simulink model "mogen_SMU_test"  (Simulink 9.2)
settings: Solver=ode4  StartTime=0.0  StopTime=6  FixedStep=model_sample_time  RelTol=1e-3
undefined symbols (not defined in the file): magnitude, model_sample_time
libraries: utils x4, simulink x2
(part 2 of 3)

== matlab function move2pose1/p2p/Cartesian_ipol2/rotation/Embedded MATLAB Function1 ==
  data: t input double; qd output double; s0 input double; v0 input double; sf input double; vm input double; am input double; dqd output double; ddqd output double; ipol_finished output double; T_scale input double; interpoly input double
function [qd,dqd,ddqd, ipol_finished] = calc_qd(t,s0,v0,sf,vm,am,T_scale,interpoly)
% This function calculates a one dimensional movement with a trapezodial 
% signal for velocity over time. Additionally it is able to adapt to shifts
% in the maximum allowed velocity.
%
% Inputs:
% t         current runtime
% s0        start value for motion in position
% v0        start value for motion in velocity
% sf        final value for motion in position
% vm        maximum allowed velocity
% am        maximum allowed acceleration
% T_scale   Scaling factor for duration of adaption
% interpoly Which interpolation to use
%
% Outputs:
% qd        disered position at current time
% dqd       disered velocity at current time
% ddqd      disered acceleration at current time
% ipol_finished 
%           motion is finished

%% Initialize persistent variables for adaption motion
persistent vm1 adpt ti qi qf T t_shift
if isempty(vm1)
    vm1 = vm;       %remembers the max velocity from last run
end
if isempty(adpt)
    adpt = false;   %stores if an adaption motion is activated
end
if isempty(ti)
    ti = 0;         %Initial time step for adaption motion
end
if isempty(qi)
    qi = zeros(3,1);%Initial values (pos,vel,acc) for adaption motion
end
if isempty(qf)
    qf = zeros(3,1);%Final values (pos,vel,acc) for adaption motion
end
if isempty(T)
    T = 0;          %Duration of adaption motion; tf = ti+T
end
if isempty(t_shift)
    t_shift = 0;    %Time distance with which the current reference motion is shifted
end

%% This If runs only for one timestep!!!
% If current max velocity is unequal to old one 
% Not directly at the beginning
% Dont start new while a adaption is still running, to prevent reset of
%   initial values
if abs(vm-vm1)>1e-3 && t>0.001 && adpt==false                       
    adpt=true;          % Activate adaption
    ti=t;               % Set initial timestep to current step

    %%% inital set of position, velo, acceleration for adaption motion 
    % is the same as the old mogen would do (t_shift is not updated at
    % this time!)
    [qi, ~] = interpolator(ti+t_shift, compute_traj_parameters(s0, v0, sf, vm1, am));

    %%% computes the time shift for shifting the new motion to the end
    % point of the old motion. So at which time the new motion has
    % the same qd? Then calculate the time distance to the inital
    % time of the change in velocities
    % t_shift < 0 if new motion is faster (vm>vm1)
    % t_shift > 0 if new motion is slower (vm<vm1)
    % interpolator_1 is the inverse function of interpolator!
    t_shift = interpolator_1(qi(1), compute_traj_parameters(s0, v0, sf, vm, am)) - ti ;

    %%% Additional shift for adaption motion = Duration of adaption motion 
    switch interpoly
        case 0
            T=0;
            adpt=false;         %no adatption  
        case 1
            T = (vm/am)*1.5;    %tanhlog
        case 2
            T = (pi*abs(qi(2)-vm))/(2*am);  %Cosine version
        case 3
            T = (vm/am);        %poly3
        case 4
            T = 1.5*(abs(qi(2)-vm)/am); %poly4
        case 5
            T = (vm/am);        %poly5 
        otherwise
            T = (vm/am);        %rest
    end

    % Scale Duration if needed
    T = T*T_scale;

    %%% The additional shift for adaption motion is dependent on the
    % difference in the velocities. See report for details.
    t_shift  = t_shift+(T/2)*((vm1/vm)-1);

    %%% Calculate final values for adaption motion. Which are reached
    % at inital time plus duration of adaption and new time shift
    [qf, ~] = interpolator(ti+T+t_shift, compute_traj_parameters(s0, v0, sf, vm, am));

end

%% Here the actual motion is calculated
% Interpolates the values of pos,vel,acc (qv) with parameters and current time t    
[qdv, ipol_finished] =interpolator(t+t_shift, compute_traj_parameters(s0, v0, sf, vm, am));  

%% If adaption motion needed
if adpt == true 

    %%% calculate the adaption moition, which takes time from ti to
    % ti+T. t is the current runtime, _i initial values, _f final
    % values, _m maximum values

    switch interpoly
        case 0
            adpt=false;                             %no adatption  
        case 1
            qdv = tanhlog(t,ti,T,qi,qf,vm,am);      %tanhlog
        case 2
            qdv = cosine(t,ti,T,qi,qf,vm,am);       %Cosine version
        case 3
            qdv = poly3(t,ti,T,qi,qf,vm,am);        %poly3
        case 4
            qdv = poly4(t,ti,T,qi,qf,vm,am);        %poly4
        case 5
            qdv = poly5(t,ti,T,qi,qf,vm,am);        %poly5 
        case 6
            qdv = poly6(t,ti,T,qi,qf,vm,am);        %poly6 
        case 7
            qdv = poly4_mean(t,ti,T,qi,qf,vm,am);   %poly4_mean 
        case 8
            qdv = poly5_2mean(t,ti,T,qi,qf,vm,am);  %poly5_2mean 
        case 9
            qdv = tanhmean(t,ti,T,qi,qf,vm,am);     %tanhmean 
        otherwise
            error('Unknown adaption motion');       %rest
    end

    %if time is equal than the finish time => adaption motion is complete
    %But it is aborted one timestep earlier, since the finish timestep
    %is already computed correctly by the standard interpolator.
    if t>=(ti+T-0.001)  %Has to be finished a bit earlier, due to errors at end
        adpt=false;     %If adaption finished => reset
    end
end

%% Set output
if sf==s0          % No motion needed if start = end 
    qd = s0;       % => set initial values
    dqd = v0;
    ddqd= 0;  
else     
    qd = qdv(1);   % set output
    dqd = qdv(2);
    ddqd = qdv(3);        
end

vm1 = vm;  %remember current max velocity

end

function [qv] = poly3(t,ti,T,qvi,qvf,dqm,ddqm)
%POLY3 computes a polynomial trajectory of degree 3 between initial (_i) 
%values and final (_f) values of position q, velocity dq and accelerataion
%ddq. Taken from Melchiorri presentation page 19

qi = qvi(1);      %split input vectors in pos,vel,acc
dqi = qvi(2);
ddqi = qvi(3);
qf = qvf(1);
dqf = qvf(2);
ddqf = qvf(3);
      
% current duration of motion dt
dt = t-ti;                      

% compute coefficients
a0 = qi;
a1 = dqi;
a2 = (-3*(qi-qf)-(2*dqi+dqf)*T)/(T^2);
a3 = (2*(qi-qf)+(dqi+dqf)*T)/(T^3);

% compute pos,vel,acc desired (_d)
qd = a0+a1*dt+a2*dt^2+a3*dt^3;
dqd = a1+2*a2*dt+3*a3*dt^2;
ddqd = 2*a2+6*a3*dt;

qv = [qd;dqd;ddqd]; %Send values back

end

function [qv] = poly4(t,ti,T,qvi,qvf,dqm,ddqm)
%POLY4 computes a polynomial trajectory of degree 4 between initial (_i) 
%values and final (_f) values of position q, velocity dq and accelerataion
%ddq. inspired by old function in here

qi = qvi(1);      %split input vectors in pos,vel,acc
dqi = qvi(2);
ddqi = qvi(3);
qf = qvf(1);
dqf = qvf(2);
ddqf = qvf(3);
      
% current duration of motion dt
dt = t-ti;                      

% a2 = 0;
% a3 = -4/9*ddqm^2/(dqi-dqm);
% a4 = -4/27*ddqm^3/(dqi-dqm)^2;
a2 = 0;
a3 = -4/9*ddqm^2/abs(dqi-dqf);
a4 = 4/27*ddqm^3/abs(dqi-dqf)^2;

a0 = qi;
a1 = dqi;
% a2 = 0.5*ddqi;
% a3 = (4*(qf-qi)-(dqf+3*dqi)*T-ddqi*(T^2))/(T^3);
% a4 = (3*(qi-qf)+(dqf+2*dqi)*T+0.5*ddqi*(T^2))/(T^4);

% compute pos,vel,acc desired (_d)
qd = (a4*dt^4+a3*dt^3+a2*dt^2+a1*dt+a0);
dqd = 4*a4*dt^3+3*a3*dt^2+2*a2*dt+a1;
ddqd = 12*a4*dt^2+6*a3*dt+2*a2;

qv = [qd;dqd;ddqd]; %Send values back

end

function [qv] = poly4_mean(t,ti,T,qvi,qvf,dqm,ddqm)
%POLY4 computes a polynomial trajectory of degree 4 between initial (_i) 
%values and final (_f) values of position q, velocity dq and accelerataion
%ddq with mean velocity at T/2. self made

qi = qvi(1);      %split input vectors in pos,vel,acc
dqi = qvi(2);
ddqi = qvi(3);
qf = qvf(1);
dqf = qvf(2);
ddqf = qvf(3);
      
% current duration of motion dt
dt = t-ti;                     

b = [qi dqi qf dqf 0.5*(dqi+dqf)]';

M_inv = [...
       1,     0,      0,          0,           0;
       0,     1,      0,          0,           0;
   6/T^2,  -2/T, -6/T^2,    5/(4*T),    27/(4*T);
 -16/T^3, 1/T^2, 16/T^3, -7/(2*T^2), -27/(2*T^2);
   9/T^4,     0, -9/T^4,  9/(4*T^3),  27/(4*T^3)];

a = M_inv * b;

% compute pos,vel,acc desired (_d)

qd = a(1)+a(2)*dt+a(3)*dt^2+a(4)*dt^3+a(5)*dt^4;
dqd = a(2)+2*a(3)*dt+3*a(4)*dt^2+4*a(5)*dt^3;
ddqd = 2*a(3)+6*a(4)*dt+12*a(5)*dt^2;

qv = [qd;dqd;ddqd]; %Send values back

end

function [qv] = poly5(t,ti,T,qvi,qvf,dqm,ddqm)
%POLY5 computes a polynomial trajectory of degree 5 between initial (_i) 
%values and final (_f) values of position q, velocity dq and accelerataion
%ddq. Taken from Melchiorri presentation page 25

qi = qvi(1);      %split input vectors in pos,vel,acc
dqi = qvi(2);
ddqi = qvi(3);
qf = qvf(1);
dqf = qvf(2);
ddqf = qvf(3);
      
% current duration of motion dt
dt = t-ti;                      

% compute coefficients
a0 = qi;
a1 = dqi;
a2 = 0.5*ddqi;
a3 = (20*(qf-qi)-(8*dqf+12*dqi)*T-(3*ddqf-ddqi)*T^2)/(2*T^3);
a4 = (30*(qi-qf)+(14*dqf+16*dqi)*T+(3*ddqf-2*ddqi)*T^2)/(2*T^4);
a5 = (12*(qf-qi)-6*(dqf+dqi)*T-(ddqf-ddqi)*T^2)/(2*T^5);

% compute pos,vel,acc desired (_d)
qd = a0+a1*dt+a2*dt^2+a3*dt^3+a4*dt^4+a5*dt^5;
dqd = a1+2*a2*dt+3*a3*dt^2+4*a4*dt^3+5*a5*dt^4;
ddqd = 2*a2+6*a3*dt+12*a4*dt^2+20*a5*dt^3;

qv = [qd;dqd;ddqd]; %Send values back

end

function [qv] = poly5_2mean(t,ti,T,qvi,qvf,dqm,ddqm)
%POLY5 computes a polynomial trajectory of degree 5 between initial (_i) 
%values and final (_f) values of position q, velocity dq and accelerataion
%ddq with 2*mean steps at T/3 and 2T/3. self made

qi = qvi(1);      %split input vectors in pos,vel,acc
dqi = qvi(2);
ddqi = qvi(3);
qf = qvf(1);
dqf = qvf(2);
ddqf = qvf(3);
      
% current duration of motion dt
dt = t-ti;                      

% compute coefficients
b = [qi dqi qf dqf 0.5*(dqi+dqf)+(1/6)*(dqi-dqf) 0.5*(dqi+dqf)+(1/6)*(dqi-dqf)]';

M_inv = [...
        1,          0,        0,           0,            0,           0;
        0,          1,        0,           0,            0,           0;
  -30/T^2,  -13/(2*T),   30/T^2,   -13/(4*T),    -27/(4*T),   -27/(2*T);
  110/T^3, 67/(4*T^2), -110/T^3,  49/(4*T^2),  135/(4*T^2), 189/(4*T^2);
 -135/T^4,    -18/T^3,  135/T^4, -63/(4*T^3), -189/(4*T^3),     -54/T^3;
   54/T^5, 27/(4*T^4),  -54/T^5,  27/(4*T^4),   81/(4*T^4),  81/(4*T^4)];

a = M_inv * b;

% compute pos,vel,acc desired (_d)

qd = a(1)+a(2)*dt+a(3)*dt^2+a(4)*dt^3+a(5)*dt^4+a(6)*dt^5;
dqd = a(2)+2*a(3)*dt+3*a(4)*dt^2+4*a(5)*dt^3+5*a(6)*dt^4;
ddqd = 2*a(3)+6*a(4)*dt+12*a(5)*dt^2+20*a(6)*dt^3;

qv = [qd;dqd;ddqd]; %Send values back

end

function [qv] = poly6(t,ti,T,qvi,qvf,dqm,ddqm)
%POLY6 computes a polynomial trajectory of degree 6 between initial (_i) 
%values and final (_f) values of position q, velocity dq and accelerataion
%ddq with mean velocity at T/3. self made

qi = qvi(1);      %split input vectors in pos,vel,acc
dqi = qvi(2);
ddqi = qvi(3);
qf = qvf(1);
dqf = qvf(2);
ddqf = qvf(3);

% current duration of motion dt
dt = t-ti;                      

% compute coefficients
b = [qi dqi 0.5*ddqi qf dqf ddqf 0.5*(dqi+dqf)]';

M_inv = [...
       1,      0,      0,       0,           0,          0,            0;
       0,      1,      0,       0,           0,          0,            0;
       0,      0,      1,       0,           0,          0,            0;
  20/T^3, -6/T^2,   -4/T, -20/T^3,  23/(4*T^2),   -1/(2*T),   81/(4*T^2);
 -75/T^4,  8/T^3,  6/T^2,  75/T^4, -89/(4*T^3),      2/T^2, -243/(4*T^3);
  84/T^5, -3/T^4, -4/T^3, -84/T^5, 105/(4*T^4), -5/(2*T^3),  243/(4*T^4);
 -30/T^6,      0,  1/T^4,  30/T^6, -39/(4*T^5),      1/T^4,  -81/(4*T^5)];

a = M_inv * b;

% compute pos,vel,acc desired (_d)

qd = a(1)+a(2)*dt+a(3)*dt^2+a(4)*dt^3+a(5)*dt^4+a(6)*dt^5+a(7)*dt^6;
dqd = a(2)+2*a(3)*dt+3*a(4)*dt^2+4*a(5)*dt^3+5*a(6)*dt^4+6*a(7)*dt^5;
ddqd = 2*a(3)+6*a(4)*dt+12*a(5)*dt^2+20*a(6)*dt^3+30*a(7)*dt^4;

qv = [qd;dqd;ddqd]; %Send values back

end

function [qv] = cosine(t,ti,T,qvi,qvf,dqm,ddqm)
%COSINE computes a cosine trajectory between initial (_i) 
%values and final (_f) values of position q, velocity dq and accelerataion
%ddq with respect to the maximum values (_m). t is the current runtime

qi = qvi(1);      %split input vectors in pos,vel,acc
dqi = qvi(2);
ddqi = qvi(3);
qf = qvf(1);
dqf = qvf(2);
ddqf = qvf(3);
      
% often needed values

%T = (pi*abs(dqf-dqi))/(2*ddqm); % total duration of motion T (with am)
%T = abs((2*(qf-qi))/(dqi-dqf));
dt = t-ti;                      % current duration of motion dt

%cm = (T/(2*pi))*(dqm-(1/T)*(qf-qi));
c = qi-0.5*(dqi+dqf)*ti;
%cn = qf-0.5*(dqi+dqf)*(ti+T);
%c = cn + 0.5*(1+cos((pi/T)*dt))*(ca-cn);


% if t<(ti+(T/2))
%     c = qi - 0.5*(dqi+dqf)*ti;
% else
%     c = qf - 0.5*(((dqi+dqf)/2)+dqf)*tf;
% end

%c = (qi+qf)/2 - 0.5*(dqi+dqf)*(ti+(T/2)) - 0.5*(dqi-dqf)*(T/pi);
% compute pos,vel,acc desired (_d)
%qd = qi + (1/T)*(qf-qi)*dt + cm*sin(((2*pi)/T)*dt);
qd = 0.5*(dqi+dqf)*t + 0.5*(T/pi)*(dqi-dqf)*sin((pi/T)*dt) + c;
dqd = 0.5*(dqi+dqf) + 0.5*(dqi-dqf)*cos((pi/T)*dt);
ddqd = -0.5*(pi/T)*(dqi-dqf)*sin((pi/T)*dt);

qv = [qd;dqd;ddqd]; %Send values back

end

function [qv] = tanhmean(t,ti,T,qvi,qvf,dqm,ddqm)
%TANHMEAN computes a tanh trajectory between initial (_i) 
%values and final (_f) values of position q, velocity dq and accelerataion
%ddq with respect to the maximum values (_m). t is the current runtime
%selfmade

qi = qvi(1);      %split input vectors in pos,vel,acc
dqi = qvi(2);
ddqi = qvi(3);
qf = qvf(1);
dqf = qvf(2);
ddqf = qvf(3);
      
% current duration of motion dt
dt = t-ti;                      
t_norm = dt/T;
theta = 4;

qd = 0.5*(1/theta)*(dqf-dqi)*log(cosh(theta*(t_norm-0.5))) ...
     + 0.5*(dqi+dqf)*t_norm ...
     + qf - 0.5*(1/theta)*(dqf-dqi)*log(cosh(0.5*theta));
     %+ qi - 0.5*(1/theta)*(dqf-dqi)*log(cosh(-0.5*theta));
dqd = 0.5*(dqi+dqf) + 0.5*(dqf-dqi)*tanh(theta*(t_norm-0.5));
ddqd = 0.5*theta*(dqf-dqi)*sech(t_norm-0.5)^2;

qv = [qd;dqd;ddqd]; %Send values back

end

function [qv] = tanhlog(t,ti,T,qvi,qvf,dqm,ddqm)
%TANHLOG computes a tanh-log trajectory between initial (_i) 
%values and final (_f) values of position q, velocity dq and accelerataion
%ddq with respect to the maximum values (_m). t is the current runtime
%taken from Internet

qi = qvi(1);      %split input vectors in pos,vel,acc
dqi = qvi(2);
ddqi = qvi(3);
qf = qvf(1);
dqf = qvf(2);
ddqf = qvf(3);
      
% current duration of motion dt
dt = t-ti;                      

a = dqi;
b = qi;      
c = dqf;
d = qf-dqf*T;
k = d-b;

x = (a*dt+b-c*dt-d+k)/(2*k);
w = (tanh(((log(1-x))^2-(log(x))^2)/3)+1)/2;
p = tanh((log(2-x)-log(x))*(1-(1/sqrt(2))*(log(2-x)+log(x))))+2*x-1;
q = tanh((log(x+1)-log(1-x))*(1-(1/sqrt(2))*(log(1-x)+log(x+1))));
s = p*(1-w)+q*w;

qd = k*s+c*dt+d-k;
dqd=(3*((tanh(((2^(1/2)*(log((10*dt)/3) + log(2 - (10*dt)/3)))/2 - 1)*(log((10*dt)/3) - log(2 - (10*dt)/3)))^2 - 1)*(((2^(1/2)*(log((10*dt)/3) + log(2 - (10*dt)/3)))/2 - 1)*(10/(3*((10*dt)/3 - 2)) - 1/dt) - (2^(1/2)*(10/(3*((10*dt)/3 - 2)) + 1/dt)*(log((10*dt)/3) - log(2 - (10*dt)/3)))/2) + 20/3)*(tanh(log((10*dt)/3)^2/3 - log(1 - (10*dt)/3)^2/3)/2 + 1/2))/100 - (3*((2*log((10*dt)/3))/(3*dt) - (20*log(1 - (10*dt)/3))/(9*((10*dt)/3 - 1)))*(tanh(log((10*dt)/3)^2/3 - log(1 - (10*dt)/3)^2/3)^2 - 1)*((20*dt)/3 + tanh(((2^(1/2)*(log((10*dt)/3) + log(2 - (10*dt)/3)))/2 - 1)*(log((10*dt)/3) - log(2 - (10*dt)/3))) - 1))/200 + (3*(tanh(((2^(1/2)*(log(1 - (10*dt)/3) + log((10*dt)/3 + 1)))/2 - 1)*(log(1 - (10*dt)/3) - log((10*dt)/3 + 1)))^2 - 1)*((10/(3*((10*dt)/3 - 1)) - 10/(3*((10*dt)/3 + 1)))*((2^(1/2)*(log(1 - (10*dt)/3) + log((10*dt)/3 + 1)))/2 - 1) + (2^(1/2)*(10/(3*((10*dt)/3 - 1)) + 10/(3*((10*dt)/3 + 1)))*(log(1 - (10*dt)/3) - log((10*dt)/3 + 1)))/2)*(tanh(log((10*dt)/3)^2/3 - log(1 - (10*dt)/3)^2/3)/2 - 1/2))/100 + (3*tanh(((2^(1/2)*(log(1 - (10*dt)/3) + log((10*dt)/3 + 1)))/2 - 1)*(log(1 - (10*dt)/3) - log((10*dt)/3 + 1)))*((2*log((10*dt)/3))/(3*dt) - (20*log(1 - (10*dt)/3))/(9*((10*dt)/3 - 1)))*(tanh(log((10*dt)/3)^2/3 - log(1 - (10*dt)/3)^2/3)^2 - 1))/200 + 3/10;
ddqd=(3*((tanh(((2^(1/2)*(log((10*dt)/3) + log(2 - (10*dt)/3)))/2 - 1)*(log((10*dt)/3) - log(2 - (10*dt)/3)))^2 - 1)*(2^(1/2)*(10/(3*((10*dt)/3 - 2)) + 1/dt)*(10/(3*((10*dt)/3 - 2)) - 1/dt) - ((2^(1/2)*(log((10*dt)/3) + log(2 - (10*dt)/3)))/2 - 1)*(100/(9*((10*dt)/3 - 2)^2) - 1/dt^2) + (2^(1/2)*(100/(9*((10*dt)/3 - 2)^2) + 1/dt^2)*(log((10*dt)/3) - log(2 - (10*dt)/3)))/2) + 2*tanh(((2^(1/2)*(log((10*dt)/3) + log(2 - (10*dt)/3)))/2 - 1)*(log((10*dt)/3) - log(2 - (10*dt)/3)))*(tanh(((2^(1/2)*(log((10*dt)/3) + log(2 - (10*dt)/3)))/2 - 1)*(log((10*dt)/3) - log(2 - (10*dt)/3)))^2 - 1)*(((2^(1/2)*(log((10*dt)/3) + log(2 - (10*dt)/3)))/2 - 1)*(10/(3*((10*dt)/3 - 2)) - 1/dt) - (2^(1/2)*(10/(3*((10*dt)/3 - 2)) + 1/dt)*(log((10*dt)/3) - log(2 - (10*dt)/3)))/2)^2)*(tanh(log((10*dt)/3)^2/3 - log(1 - (10*dt)/3)^2/3)/2 + 1/2))/100 - (3*((2*log((10*dt)/3))/(3*dt) - (20*log(1 - (10*dt)/3))/(9*((10*dt)/3 - 1)))*((tanh(((2^(1/2)*(log((10*dt)/3) + log(2 - (10*dt)/3)))/2 - 1)*(log((10*dt)/3) - log(2 - (10*dt)/3)))^2 - 1)*(((2^(1/2)*(log((10*dt)/3) + log(2 - (10*dt)/3)))/2 - 1)*(10/(3*((10*dt)/3 - 2)) - 1/dt) - (2^(1/2)*(10/(3*((10*dt)/3 - 2)) + 1/dt)*(log((10*dt)/3) - log(2 - (10*dt)/3)))/2) + 20/3)*(tanh(log((10*dt)/3)^2/3 - log(1 - (10*dt)/3)^2/3)^2 - 1))/100 + (3*(tanh(log((10*dt)/3)^2/3 - log(1 - (10*dt)/3)^2/3)^2 - 1)*((20*dt)/3 + tanh(((2^(1/2)*(log((10*dt)/3) + log(2 - (10*dt)/3)))/2 - 1)*(log((10*dt)/3) - log(2 - (10*dt)/3))) - 1)*((2*log((10*dt)/3))/(3*dt^2) - (200*log(1 - (10*dt)/3))/(27*((10*dt)/3 - 1)^2) + 200/(27*((10*dt)/3 - 1)^2) - 2/(3*dt^2)))/200 - (3*(tanh(((2^(1/2)*(log(1 - (10*dt)/3) + log((10*dt)/3 + 1)))/2 - 1)*(log(1 - (10*dt)/3) - log((10*dt)/3 + 1)))^2 - 1)*(tanh(log((10*dt)/3)^2/3 - log(1 - (10*dt)/3)^2/3)/2 - 1/2)*((100/(9*((10*dt)/3 - 1)^2) - 100/(9*((10*dt)/3 + 1)^2))*((2^(1/2)*(log(1 - (10*dt)/3) + log((10*dt)/3 + 1)))/2 - 1) - 2^(1/2)*(10/(3*((10*dt)/3 - 1)) - 10/(3*((10*dt)/3 + 1)))*(10/(3*((10*dt)/3 - 1)) + 10/(3*((10*dt)/3 + 1))) + (2^(1/2)*(100/(9*((10*dt)/3 - 1)^2) + 100/(9*((10*dt)/3 + 1)^2))*(log(1 - (10*dt)/3) - log((10*dt)/3 + 1)))/2))/100 - (3*tanh(((2^(1/2)*(log(1 - (10*dt)/3) + log((10*dt)/3 + 1)))/2 - 1)*(log(1 - (10*dt)/3) - log((10*dt)/3 + 1)))*(tanh(log((10*dt)/3)^2/3 - log(1 - (10*dt)/3)^2/3)^2 - 1)*((2*log((10*dt)/3))/(3*dt^2) - (200*log(1 - (10*dt)/3))/(27*((10*dt)/3 - 1)^2) + 200/(27*((10*dt)/3 - 1)^2) - 2/(3*dt^2)))/200 - (3*tanh(log((10*dt)/3)^2/3 - log(1 - (10*dt)/3)^2/3)*tanh(((2^(1/2)*(log(1 - (10*dt)/3) + log((10*dt)/3 + 1)))/2 - 1)*(log(1 - (10*dt)/3) - log((10*dt)/3 + 1)))*((2*log((10*dt)/3))/(3*dt) - (20*log(1 - (10*dt)/3))/(9*((10*dt)/3 - 1)))^2*(tanh(log((10*dt)/3)^2/3 - log(1 - (10*dt)/3)^2/3)^2 - 1))/100 - (3*tanh(((2^(1/2)*(log(1 - (10*dt)/3) + log((10*dt)/3 + 1)))/2 - 1)*(log(1 - (10*dt)/3) - log((10*dt)/3 + 1)))*(tanh(((2^(1/2)*(log(1 - (10*dt)/3) + log((10*dt)/3 + 1)))/2 - 1)*(log(1 - (10*dt)/3) - log((10*dt)/3 + 1)))^2 - 1)*((10/(3*((10*dt)/3 - 1)) - 10/(3*((10*dt)/3 + 1)))*((2^(1/2)*(log(1 - (10*dt)/3) + log((10*dt)/3 + 1)))/2 - 1) + (2^(1/2)*(10/(3*((10*dt)/3 - 1)) + 10/(3*((10*dt)/3 + 1)))*(log(1 - (10*dt)/3) - log((10*dt)/3 + 1)))/2)^2*(tanh(log((10*dt)/3)^2/3 - log(1 - (10*dt)/3)^2/3)/2 - 1/2))/50 + (3*tanh(log((10*dt)/3)^2/3 - log(1 - (10*dt)/3)^2/3)*((2*log((10*dt)/3))/(3*dt) - (20*log(1 - (10*dt)/3))/(9*((10*dt)/3 - 1)))^2*(tanh(log((10*dt)/3)^2/3 - log(1 - (10*dt)/3)^2/3)^2 - 1)*((20*dt)/3 + tanh(((2^(1/2)*(log((10*dt)/3) + log(2 - (10*dt)/3)))/2 - 1)*(log((10*dt)/3) - log(2 - (10*dt)/3))) - 1))/100 - (3*(tanh(((2^(1/2)*(log(1 - (10*dt)/3) + log((10*dt)/3 + 1)))/2 - 1)*(log(1 - (10*dt)/3) - log((10*dt)/3 + 1)))^2 - 1)*((2*log((10*dt)/3))/(3*dt) - (20*log(1 - (10*dt)/3))/(9*((10*dt)/3 - 1)))*((10/(3*((10*dt)/3 - 1)) - 10/(3*((10*dt)/3 + 1)))*((2^(1/2)*(log(1 - (10*dt)/3) + log((10*dt)/3 + 1)))/2 - 1) + (2^(1/2)*(10/(3*((10*dt)/3 - 1)) + 10/(3*((10*dt)/3 + 1)))*(log(1 - (10*dt)/3) - log((10*dt)/3 + 1)))/2)*(tanh(log((10*dt)/3)^2/3 - log(1 - (10*dt)/3)^2/3)^2 - 1))/100;

qv = [qd;dqd;ddqd]; %Send values back

end

function ris=compute_traj_parameters(s0, v0, sf, vm, am)
    ris=zeros(15,1);
    radix=zeros(2,1);
    T1 = 0;
    dT = 0;
    T2 = 0;
    a1 = 0;
    b1 = 0;
    c1 = 0;
    d1 = 0;
    e1 = 0;
    a2 = 0;
    b2 = 0;
    c2 = 0;
    d2 = 0;
    e2 = 0;
    k = 0;

    if (vm~=0) %check...
        vm=vm*sign(sf-s0);
        k=am*sign(sf-s0);
        T1 = -3/2*(v0-vm)/k;
        a1 = -4/27*k^3/(v0-vm)^2;
        b1 = -4/9*k^2/(v0-vm);
        e1 = s0;
        d1 = v0;
        c1 = 0;
        c2 = 0;
        T2 = 3/2*vm/k;
        dT = 1/4*(-3*vm^2+4*sf*k-4*a1*T1^4*k-4*b1*T1^3*k-4*c1*T1^2*k-4*d1*T1*k-4*e1*k)/vm/k;
        a2 = 4/27*k^3/vm^2;
        d2 = vm;
        e2 = 1/4*(-3*vm^2+4*sf*k)/k;
        b2 = -4/9*k^2/vm;
        if (dT<0)
            c2 = 0;
            c1 = 0;
            a=2;
            b=12*v0;
            c=9*v0^2-12*sf*k+12*s0*k;
            radix(1)=(-b + sqrt(b^2-4*a*c))/(2*a);
            radix(2)=(-b - sqrt(b^2-4*a*c))/(2*a);
            %decide the correct root
            T1_a = 1/2*radix(1)/k;
            T2_a = 1/2*(radix(1)+3*v0)/k;
            T1_b = 1/2*radix(2)/k;
            T2_b = 1/2*(radix(2)+3*v0)/k;
                if (and(T1_a>=0, T2_a>=0))
                    r=radix(1);
                    T1=T1_a;
                    T2=T2_a;
                    dT=0;
                    two_phases=1;
                elseif (and(T1_b>=0, T2_b>=0))
                    r=radix(2);
                    T1=T1_b;
                    T2=T2_b;
                    dT=0;
                    two_phases=1;
                else
                    r=0;
                    two_phases=0;
                end
                if (two_phases==0)
                    T1=0;
                    T2=2*(sf-s0)/v0;
                    dT=0;
                    b2=-1/4*v0^3/(sf-s0)^2;
                    c2=0;
                    a2=1/16*v0^4/(sf-s0)^3;
                    d2=v0;
                    e2=s0;
                else
                    b1 = -8/9*k^2/(4*v0*r+3*v0^2-4*sf*k+4*s0*k)*r;
                    a1 = 8/9*k^3/(4*v0*r+3*v0^2-4*sf*k+4*s0*k);
                    b2 = -8/9*k^2/(4*sf*k+3*v0^2-4*s0*k)*(r+3*v0);
                    e2 = -1/8*(3*v0^2-4*s0*k-4*sf*k)/k;
                    e1 = s0;
                    d1 = v0;
                    d2 = 2/9/(4*sf*k+3*v0^2-4*s0*k)*(r+3*v0)^3;
                    a2 = 8/9*k^3/(4*sf*k+3*v0^2-4*s0*k);
                end
        end
    end
    ris=[T1;dT;T2; a1; b1; c1; d1; e1; a2; b2; c2; d2; e2; vm; k];
end

%time, and the output of the previous function
function [ris, finished]=interpolator(t, parameters)

ris=zeros(3,1);
T1=parameters(1);
dT=parameters(2);
T2=parameters(3);
a1=parameters(4);
b1=parameters(5);
c1=parameters(6);
d1=parameters(7);
e1=parameters(8);
a2=parameters(9);
b2=parameters(10);
c2=parameters(11);
d2=parameters(12);
e2=parameters(13);
vm=parameters(14);
k=parameters(15);

finished = 0;
if (vm~=0) %check...
        if (t<=T1)
            ris=[a1*t^4+b1*t^3+c1*t^2+d1*t+e1; 4*a1*t^3+3*b1*t^2+2*c1*t+d1; 12*a1*t^2+6*b1*t+2*c1];
        elseif (t<=T1+dT)
            t=t-T1;
            ris=[a1*T1^4+b1*T1^3+c1*T1^2+d1*T1+e1+vm*t; vm; 0];
        elseif (t<=T1+dT+T2)
            t=t-T1-dT;
            ris=[a2*t^4+b2*t^3+c2*t^2+d2*t+e2; 4*a2*t^3+3*b2*t^2+2*c2*t+d2; 12*a2*t^2+6*b2*t+2*c2];
        else
            t=T2;
            ris=[a2*t^4+b2*t^3+c2*t^2+d2*t+e2;0;0];
            finished=1;
        end
else
    ris=[0;0;0];
end

end

function t=interpolator_1(q, parameters)

T1=parameters(1);
dT=parameters(2);
T2=parameters(3);
a1=parameters(4);
b1=parameters(5);
c1=parameters(6);
d1=parameters(7);
e1=parameters(8);
a2=parameters(9);
b2=parameters(10);
c2=parameters(11);
d2=parameters(12);
e2=parameters(13);
vm=parameters(14);
k=parameters(15);

t=0;
Q1 = a1*T1^4+b1*T1^3+c1*T1^2+d1*T1+e1;%q point at end of startup
Q2 = a2*T2^4+b2*T2^3+c2*T2^2+d2*T2+e2;%final q
Q3 = Q2-Q1;%q point at end of linear part (using symmetry)

if q<Q1
    %startup
%     %tarray = 0:0.001:T1; %not working, because T1 should be constant?!
%     tarray = linspace(0,T1);
%     qarray=zeros(size(tarray));
%     parfor i=1:size(tarray,2)
%         [qv,~]=interpolator(tarray(i), parameters);
%         qarray(i)=qv(1);
%     end
%     t = interp1(qarray, tarray, q);
    t=0;
    error('trans: interpolator_1 startup: not programmed jet, sry');
    % problem with calculating additional shift
elseif q>=Q1 || q<=Q3
    %linear part
    t = T1+((q-Q1)/vm);
elseif q>Q3
    %slowdown
    t=0;
    error('trans: interpolator_1 slowdown: not programmed jet, sry');
end

end

== matlab function move2pose1/p2p/Cartesian_ipol2/translation/Embedded MATLAB Function1 ==
  data: t input double; qd output double; s0 input double; v0 input double; sf input double; vm input double; am input double; dqd output double; ddqd output double; ipol_finished output double; T_scale input double; interpoly input double
function [qd,dqd,ddqd, ipol_finished] = calc_qd(t,s0,v0,sf,vm,am,T_scale,interpoly)
% This function calculates a one dimensional movement with a trapezodial 
% signal for velocity over time. Additionally it is able to adapt to shifts
% in the maximum allowed velocity.
%
% Inputs:
% t         current runtime
% s0        start value for motion in position
% v0        start value for motion in velocity
% sf        final value for motion in position
% vm        maximum allowed velocity
% am        maximum allowed acceleration
% T_scale   Scaling factor for duration of adaption
% interpoly Which interpolation to use
%
% Outputs:
% qd        disered position at current time
% dqd       disered velocity at current time
% ddqd      disered acceleration at current time
% ipol_finished 
%           motion is finished

%% Initialize persistent variables for adaption motion
persistent vm1 adpt ti qi qf T t_shift
if isempty(vm1)
    vm1 = vm;       %remembers the max velocity from last run
end
if isempty(adpt)
    adpt = false;   %stores if an adaption motion is activated
end
if isempty(ti)
    ti = 0;         %Initial time step for adaption motion
end
if isempty(qi)
    qi = zeros(3,1);%Initial values (pos,vel,acc) for adaption motion
end
if isempty(qf)
    qf = zeros(3,1);%Final values (pos,vel,acc) for adaption motion
end
if isempty(T)
    T = 0;          %Duration of adaption motion; tf = ti+T
end
if isempty(t_shift)
    t_shift = 0;    %Time distance with which the current reference motion is shifted
end

%% This If runs only for one timestep!!!
% If current max velocity is unequal to old one 
% Not directly at the beginning
% Dont start new while a adaption is still running, to prevent reset of
%   initial values
if abs(vm-vm1)>1e-3 && t>0.001 && adpt==false                       
    adpt=true;          % Activate adaption
    ti=t;               % Set initial timestep to current step

    %%% inital set of position, velo, acceleration for adaption motion 
    % is the same as the old mogen would do (t_shift is not updated at
    % this time!)
    [qi, ~] = interpolator(ti+t_shift, compute_traj_parameters(s0, v0, sf, vm1, am));

    %%% computes the time shift for shifting the new motion to the end
    % point of the old motion. So at which time the new motion has
    % the same qd? Then calculate the time distance to the inital
    % time of the change in velocities
    % t_shift < 0 if new motion is faster (vm>vm1)
    % t_shift > 0 if new motion is slower (vm<vm1)
    % interpolator_1 is the inverse function of interpolator!
    t_shift = interpolator_1(qi(1), compute_traj_parameters(s0, v0, sf, vm, am)) - ti ;

    %%% Additional shift for adaption motion = Duration of adaption motion 
    switch interpoly
        case 0
            T=0;
            adpt=false;         %no adatption  
        case 1
            T = (vm/am)*1.5;    %tanhlog
        case 2
            T = (pi*abs(qi(2)-vm))/(2*am);  %Cosine version
        case 3
            T = (vm/am);        %poly3
        case 4
            T = 1.5*(abs(qi(2)-vm)/am); %poly4
        case 5
            T = (vm/am);        %poly5 
        otherwise
            T = (vm/am);        %rest
    end

    % Scale Duration if needed
    T = T*T_scale;

    %%% The additional shift for adaption motion is dependent on the
    % difference in the velocities. See report for details.
    t_shift  = t_shift+(T/2)*((vm1/vm)-1);

    %%% Calculate final values for adaption motion. Which are reached
    % at inital time plus duration of adaption and new time shift
    [qf, ~] = interpolator(ti+T+t_shift, compute_traj_parameters(s0, v0, sf, vm, am));

end

%% Here the actual motion is calculated
% Interpolates the values of pos,vel,acc (qv) with parameters and current time t    
[qdv, ipol_finished] =interpolator(t+t_shift, compute_traj_parameters(s0, v0, sf, vm, am));  

%% If adaption motion needed
if adpt == true 

    %%% calculate the adaption moition, which takes time from ti to
    % ti+T. t is the current runtime, _i initial values, _f final
    % values, _m maximum values

    switch interpoly
        case 0
            adpt=false;                             %no adatption  
        case 1
            qdv = tanhlog(t,ti,T,qi,qf,vm,am);      %tanhlog
        case 2
            qdv = cosine(t,ti,T,qi,qf,vm,am);       %Cosine version
        case 3
            qdv = poly3(t,ti,T,qi,qf,vm,am);        %poly3
        case 4
            qdv = poly4(t,ti,T,qi,qf,vm,am);        %poly4
        case 5
            qdv = poly5(t,ti,T,qi,qf,vm,am);        %poly5 
        case 6
            qdv = poly6(t,ti,T,qi,qf,vm,am);        %poly6 
        case 7
            qdv = poly4_mean(t,ti,T,qi,qf,vm,am);   %poly4_mean 
        case 8
            qdv = poly5_2mean(t,ti,T,qi,qf,vm,am);  %poly5_2mean 
        case 9
            qdv = tanhmean(t,ti,T,qi,qf,vm,am);     %tanhmean 
        otherwise
            error('Unknown adaption motion');       %rest
    end

    %if time is equal than the finish time => adaption motion is complete
    %But it is aborted one timestep earlier, since the finish timestep
    %is already computed correctly by the standard interpolator.
    if t>=(ti+T-0.001)  %Has to be finished a bit earlier, due to errors at end
        adpt=false;     %If adaption finished => reset
    end
end

%% Set output
if sf==s0          % No motion needed if start = end 
    qd = s0;       % => set initial values
    dqd = v0;
    ddqd= 0;  
else     
    qd = qdv(1);   % set output
    dqd = qdv(2);
    ddqd = qdv(3);        
end

vm1 = vm;  %remember current max velocity

end

function [qv] = poly3(t,ti,T,qvi,qvf,dqm,ddqm)
%POLY3 computes a polynomial trajectory of degree 3 between initial (_i) 
%values and final (_f) values of position q, velocity dq and accelerataion
%ddq. Taken from Melchiorri presentation page 19

qi = qvi(1);      %split input vectors in pos,vel,acc
dqi = qvi(2);
ddqi = qvi(3);
qf = qvf(1);
dqf = qvf(2);
ddqf = qvf(3);
      
% current duration of motion dt
dt = t-ti;                      

% compute coefficients
a0 = qi;
a1 = dqi;
a2 = (-3*(qi-qf)-(2*dqi+dqf)*T)/(T^2);
a3 = (2*(qi-qf)+(dqi+dqf)*T)/(T^3);

% compute pos,vel,acc desired (_d)
qd = a0+a1*dt+a2*dt^2+a3*dt^3;
dqd = a1+2*a2*dt+3*a3*dt^2;
ddqd = 2*a2+6*a3*dt;

qv = [qd;dqd;ddqd]; %Send values back

end

function [qv] = poly4(t,ti,T,qvi,qvf,dqm,ddqm)
%POLY4 computes a polynomial trajectory of degree 4 between initial (_i) 
%values and final (_f) values of position q, velocity dq and accelerataion
%ddq. inspired by old function in here

qi = qvi(1);      %split input vectors in pos,vel,acc
dqi = qvi(2);
ddqi = qvi(3);
qf = qvf(1);
dqf = qvf(2);
ddqf = qvf(3);
      
% current duration of motion dt
dt = t-ti;                      

% a2 = 0;
% a3 = -4/9*ddqm^2/(dqi-dqm);
% a4 = -4/27*ddqm^3/(dqi-dqm)^2;
a2 = 0;
a3 = -4/9*ddqm^2/abs(dqi-dqf);
a4 = 4/27*ddqm^3/abs(dqi-dqf)^2;

a0 = qi;
a1 = dqi;
% a2 = 0.5*ddqi;
% a3 = (4*(qf-qi)-(dqf+3*dqi)*T-ddqi*(T^2))/(T^3);
% a4 = (3*(qi-qf)+(dqf+2*dqi)*T+0.5*ddqi*(T^2))/(T^4);

% compute pos,vel,acc desired (_d)
qd = (a4*dt^4+a3*dt^3+a2*dt^2+a1*dt+a0);
dqd = 4*a4*dt^3+3*a3*dt^2+2*a2*dt+a1;
ddqd = 12*a4*dt^2+6*a3*dt+2*a2;

qv = [qd;dqd;ddqd]; %Send values back

end

function [qv] = poly4_mean(t,ti,T,qvi,qvf,dqm,ddqm)
%POLY4 computes a polynomial trajectory of degree 4 between initial (_i) 
%values and final (_f) values of position q, velocity dq and accelerataion
%ddq with mean velocity at T/2. self made

qi = qvi(1);      %split input vectors in pos,vel,acc
dqi = qvi(2);
ddqi = qvi(3);
qf = qvf(1);
dqf = qvf(2);
ddqf = qvf(3);
      
% current duration of motion dt
dt = t-ti;                     

b = [qi dqi qf dqf 0.5*(dqi+dqf)]';

M_inv = [...
       1,     0,      0,          0,           0;
       0,     1,      0,          0,           0;
   6/T^2,  -2/T, -6/T^2,    5/(4*T),    27/(4*T);
 -16/T^3, 1/T^2, 16/T^3, -7/(2*T^2), -27/(2*T^2);
   9/T^4,     0, -9/T^4,  9/(4*T^3),  27/(4*T^3)];

a = M_inv * b;

% compute pos,vel,acc desired (_d)

qd = a(1)+a(2)*dt+a(3)*dt^2+a(4)*dt^3+a(5)*dt^4;
dqd = a(2)+2*a(3)*dt+3*a(4)*dt^2+4*a(5)*dt^3;
ddqd = 2*a(3)+6*a(4)*dt+12*a(5)*dt^2;

qv = [qd;dqd;ddqd]; %Send values back

end

function [qv] = poly5(t,ti,T,qvi,qvf,dqm,ddqm)
%POLY5 computes a polynomial trajectory of degree 5 between initial (_i) 
%values and final (_f) values of position q, velocity dq and accelerataion
%ddq. Taken from Melchiorri presentation page 25

qi = qvi(1);      %split input vectors in pos,vel,acc
dqi = qvi(2);
ddqi = qvi(3);
qf = qvf(1);
dqf = qvf(2);
ddqf = qvf(3);
      
% current duration of motion dt
dt = t-ti;                      

% compute coefficients
a0 = qi;
a1 = dqi;
a2 = 0.5*ddqi;
a3 = (20*(qf-qi)-(8*dqf+12*dqi)*T-(3*ddqf-ddqi)*T^2)/(2*T^3);
a4 = (30*(qi-qf)+(14*dqf+16*dqi)*T+(3*ddqf-2*ddqi)*T^2)/(2*T^4);
a5 = (12*(qf-qi)-6*(dqf+dqi)*T-(ddqf-ddqi)*T^2)/(2*T^5);

% compute pos,vel,acc desired (_d)
qd = a0+a1*dt+a2*dt^2+a3*dt^3+a4*dt^4+a5*dt^5;
dqd = a1+2*a2*dt+3*a3*dt^2+4*a4*dt^3+5*a5*dt^4;
ddqd = 2*a2+6*a3*dt+12*a4*dt^2+20*a5*dt^3;

qv = [qd;dqd;ddqd]; %Send values back

end

function [qv] = poly5_2mean(t,ti,T,qvi,qvf,dqm,ddqm)
%POLY5 computes a polynomial trajectory of degree 5 between initial (_i) 
%values and final (_f) values of position q, velocity dq and accelerataion
%ddq with 2*mean steps at T/3 and 2T/3. self made

qi = qvi(1);      %split input vectors in pos,vel,acc
dqi = qvi(2);
ddqi = qvi(3);
qf = qvf(1);
dqf = qvf(2);
ddqf = qvf(3);
      
% current duration of motion dt
dt = t-ti;                      

% compute coefficients
b = [qi dqi qf dqf 0.5*(dqi+dqf)+(1/6)*(dqi-dqf) 0.5*(dqi+dqf)+(1/6)*(dqi-dqf)]';

M_inv = [...
        1,          0,        0,           0,            0,           0;
        0,          1,        0,           0,            0,           0;
  -30/T^2,  -13/(2*T),   30/T^2,   -13/(4*T),    -27/(4*T),   -27/(2*T);
  110/T^3, 67/(4*T^2), -110/T^3,  49/(4*T^2),  135/(4*T^2), 189/(4*T^2);
 -135/T^4,    -18/T^3,  135/T^4, -63/(4*T^3), -189/(4*T^3),     -54/T^3;
   54/T^5, 27/(4*T^4),  -54/T^5,  27/(4*T^4),   81/(4*T^4),  81/(4*T^4)];

a = M_inv * b;

% compute pos,vel,acc desired (_d)

qd = a(1)+a(2)*dt+a(3)*dt^2+a(4)*dt^3+a(5)*dt^4+a(6)*dt^5;
dqd = a(2)+2*a(3)*dt+3*a(4)*dt^2+4*a(5)*dt^3+5*a(6)*dt^4;
ddqd = 2*a(3)+6*a(4)*dt+12*a(5)*dt^2+20*a(6)*dt^3;

qv = [qd;dqd;ddqd]; %Send values back

end

function [qv] = poly6(t,ti,T,qvi,qvf,dqm,ddqm)
%POLY6 computes a polynomial trajectory of degree 6 between initial (_i) 
%values and final (_f) values of position q, velocity dq and accelerataion
%ddq with mean velocity at T/3. self made

qi = qvi(1);      %split input vectors in pos,vel,acc
dqi = qvi(2);
ddqi = qvi(3);
qf = qvf(1);
dqf = qvf(2);
ddqf = qvf(3);

% current duration of motion dt
dt = t-ti;                      

% compute coefficients
b = [qi dqi 0.5*ddqi qf dqf ddqf 0.5*(dqi+dqf)]';

M_inv = [...
       1,      0,      0,       0,           0,          0,            0;
       0,      1,      0,       0,           0,          0,            0;
       0,      0,      1,       0,           0,          0,            0;
  20/T^3, -6/T^2,   -4/T, -20/T^3,  23/(4*T^2),   -1/(2*T),   81/(4*T^2);
 -75/T^4,  8/T^3,  6/T^2,  75/T^4, -89/(4*T^3),      2/T^2, -243/(4*T^3);
  84/T^5, -3/T^4, -4/T^3, -84/T^5, 105/(4*T^4), -5/(2*T^3),  243/(4*T^4);
 -30/T^6,      0,  1/T^4,  30/T^6, -39/(4*T^5),      1/T^4,  -81/(4*T^5)];

a = M_inv * b;

% compute pos,vel,acc desired (_d)

qd = a(1)+a(2)*dt+a(3)*dt^2+a(4)*dt^3+a(5)*dt^4+a(6)*dt^5+a(7)*dt^6;
dqd = a(2)+2*a(3)*dt+3*a(4)*dt^2+4*a(5)*dt^3+5*a(6)*dt^4+6*a(7)*dt^5;
ddqd = 2*a(3)+6*a(4)*dt+12*a(5)*dt^2+20*a(6)*dt^3+30*a(7)*dt^4;

qv = [qd;dqd;ddqd]; %Send values back

end

function [qv] = cosine(t,ti,T,qvi,qvf,dqm,ddqm)
%COSINE computes a cosine trajectory between initial (_i) 
%values and final (_f) values of position q, velocity dq and accelerataion
%ddq with respect to the maximum values (_m). t is the current runtime

qi = qvi(1);      %split input vectors in pos,vel,acc
dqi = qvi(2);
ddqi = qvi(3);
qf = qvf(1);
dqf = qvf(2);
ddqf = qvf(3);
      
% often needed values

%T = (pi*abs(dqf-dqi))/(2*ddqm); % total duration of motion T (with am)
%T = abs((2*(qf-qi))/(dqi-dqf));
dt = t-ti;                      % current duration of motion dt

%cm = (T/(2*pi))*(dqm-(1/T)*(qf-qi));
c = qi-0.5*(dqi+dqf)*ti;
%cn = qf-0.5*(dqi+dqf)*(ti+T);
%c = cn + 0.5*(1+cos((pi/T)*dt))*(ca-cn);


% if t<(ti+(T/2))
%     c = qi - 0.5*(dqi+dqf)*ti;
% else
%     c = qf - 0.5*(((dqi+dqf)/2)+dqf)*tf;
% end

%c = (qi+qf)/2 - 0.5*(dqi+dqf)*(ti+(T/2)) - 0.5*(dqi-dqf)*(T/pi);
% compute pos,vel,acc desired (_d)
%qd = qi + (1/T)*(qf-qi)*dt + cm*sin(((2*pi)/T)*dt);
qd = 0.5*(dqi+dqf)*t + 0.5*(T/pi)*(dqi-dqf)*sin((pi/T)*dt) + c;
dqd = 0.5*(dqi+dqf) + 0.5*(dqi-dqf)*cos((pi/T)*dt);
ddqd = -0.5*(pi/T)*(dqi-dqf)*sin((pi/T)*dt);

qv = [qd;dqd;ddqd]; %Send values back

end

function [qv] = tanhmean(t,ti,T,qvi,qvf,dqm,ddqm)
%TANHMEAN computes a tanh trajectory between initial (_i) 
%values and final (_f) values of position q, velocity dq and accelerataion
%ddq with respect to the maximum values (_m). t is the current runtime
%selfmade

qi = qvi(1);      %split input vectors in pos,vel,acc
dqi = qvi(2);
ddqi = qvi(3);
qf = qvf(1);
dqf = qvf(2);
ddqf = qvf(3);
      
% current duration of motion dt
dt = t-ti;                      
t_norm = dt/T;
theta = 4;

qd = 0.5*(1/theta)*(dqf-dqi)*log(cosh(theta*(t_norm-0.5))) ...
     + 0.5*(dqi+dqf)*t_norm ...
     + qf - 0.5*(1/theta)*(dqf-dqi)*log(cosh(0.5*theta));
     %+ qi - 0.5*(1/theta)*(dqf-dqi)*log(cosh(-0.5*theta));
dqd = 0.5*(dqi+dqf) + 0.5*(dqf-dqi)*tanh(theta*(t_norm-0.5));
ddqd = 0.5*theta*(dqf-dqi)*sech(t_norm-0.5)^2;

qv = [qd;dqd;ddqd]; %Send values back

end

function [qv] = tanhlog(t,ti,T,qvi,qvf,dqm,ddqm)
%TANHLOG computes a tanh-log trajectory between initial (_i) 
%values and final (_f) values of position q, velocity dq and accelerataion
%ddq with respect to the maximum values (_m). t is the current runtime
%taken from Internet

qi = qvi(1);      %split input vectors in pos,vel,acc
dqi = qvi(2);
ddqi = qvi(3);
qf = qvf(1);
dqf = qvf(2);
ddqf = qvf(3);
      
% current duration of motion dt
dt = t-ti;                      

a = dqi;
b = qi;      
c = dqf;
d = qf-dqf*T;
k = d-b;

x = (a*dt+b-c*dt-d+k)/(2*k);
w = (tanh(((log(1-x))^2-(log(x))^2)/3)+1)/2;
p = tanh((log(2-x)-log(x))*(1-(1/sqrt(2))*(log(2-x)+log(x))))+2*x-1;
q = tanh((log(x+1)-log(1-x))*(1-(1/sqrt(2))*(log(1-x)+log(x+1))));
s = p*(1-w)+q*w;

qd = k*s+c*dt+d-k;
dqd=(3*((tanh(((2^(1/2)*(log((10*dt)/3) + log(2 - (10*dt)/3)))/2 - 1)*(log((10*dt)/3) - log(2 - (10*dt)/3)))^2 - 1)*(((2^(1/2)*(log((10*dt)/3) + log(2 - (10*dt)/3)))/2 - 1)*(10/(3*((10*dt)/3 - 2)) - 1/dt) - (2^(1/2)*(10/(3*((10*dt)/3 - 2)) + 1/dt)*(log((10*dt)/3) - log(2 - (10*dt)/3)))/2) + 20/3)*(tanh(log((10*dt)/3)^2/3 - log(1 - (10*dt)/3)^2/3)/2 + 1/2))/100 - (3*((2*log((10*dt)/3))/(3*dt) - (20*log(1 - (10*dt)/3))/(9*((10*dt)/3 - 1)))*(tanh(log((10*dt)/3)^2/3 - log(1 - (10*dt)/3)^2/3)^2 - 1)*((20*dt)/3 + tanh(((2^(1/2)*(log((10*dt)/3) + log(2 - (10*dt)/3)))/2 - 1)*(log((10*dt)/3) - log(2 - (10*dt)/3))) - 1))/200 + (3*(tanh(((2^(1/2)*(log(1 - (10*dt)/3) + log((10*dt)/3 + 1)))/2 - 1)*(log(1 - (10*dt)/3) - log((10*dt)/3 + 1)))^2 - 1)*((10/(3*((10*dt)/3 - 1)) - 10/(3*((10*dt)/3 + 1)))*((2^(1/2)*(log(1 - (10*dt)/3) + log((10*dt)/3 + 1)))/2 - 1) + (2^(1/2)*(10/(3*((10*dt)/3 - 1)) + 10/(3*((10*dt)/3 + 1)))*(log(1 - (10*dt)/3) - log((10*dt)/3 + 1)))/2)*(tanh(log((10*dt)/3)^2/3 - log(1 - (10*dt)/3)^2/3)/2 - 1/2))/100 + (3*tanh(((2^(1/2)*(log(1 - (10*dt)/3) + log((10*dt)/3 + 1)))/2 - 1)*(log(1 - (10*dt)/3) - log((10*dt)/3 + 1)))*((2*log((10*dt)/3))/(3*dt) - (20*log(1 - (10*dt)/3))/(9*((10*dt)/3 - 1)))*(tanh(log((10*dt)/3)^2/3 - log(1 - (10*dt)/3)^2/3)^2 - 1))/200 + 3/10;
ddqd=(3*((tanh(((2^(1/2)*(log((10*dt)/3) + log(2 - (10*dt)/3)))/2 - 1)*(log((10*dt)/3) - log(2 - (10*dt)/3)))^2 - 1)*(2^(1/2)*(10/(3*((10*dt)/3 - 2)) + 1/dt)*(10/(3*((10*dt)/3 - 2)) - 1/dt) - ((2^(1/2)*(log((10*dt)/3) + log(2 - (10*dt)/3)))/2 - 1)*(100/(9*((10*dt)/3 - 2)^2) - 1/dt^2) + (2^(1/2)*(100/(9*((10*dt)/3 - 2)^2) + 1/dt^2)*(log((10*dt)/3) - log(2 - (10*dt)/3)))/2) + 2*tanh(((2^(1/2)*(log((10*dt)/3) + log(2 - (10*dt)/3)))/2 - 1)*(log((10*dt)/3) - log(2 - (10*dt)/3)))*(tanh(((2^(1/2)*(log((10*dt)/3) + log(2 - (10*dt)/3)))/2 - 1)*(log((10*dt)/3) - log(2 - (10*dt)/3)))^2 - 1)*(((2^(1/2)*(log((10*dt)/3) + log(2 - (10*dt)/3)))/2 - 1)*(10/(3*((10*dt)/3 - 2)) - 1/dt) - (2^(1/2)*(10/(3*((10*dt)/3 - 2)) + 1/dt)*(log((10*dt)/3) - log(2 - (10*dt)/3)))/2)^2)*(tanh(log((10*dt)/3)^2/3 - log(1 - (10*dt)/3)^2/3)/2 + 1/2))/100 - (3*((2*log((10*dt)/3))/(3*dt) - (20*log(1 - (10*dt)/3))/(9*((10*dt)/3 - 1)))*((tanh(((2^(1/2)*(log((10*dt)/3) + log(2 - (10*dt)/3)))/2 - 1)*(log((10*dt)/3) - log(2 - (10*dt)/3)))^2 - 1)*(((2^(1/2)*(log((10*dt)/3) + log(2 - (10*dt)/3)))/2 - 1)*(10/(3*((10*dt)/3 - 2)) - 1/dt) - (2^(1/2)*(10/(3*((10*dt)/3 - 2)) + 1/dt)*(log((10*dt)/3) - log(2 - (10*dt)/3)))/2) + 20/3)*(tanh(log((10*dt)/3)^2/3 - log(1 - (10*dt)/3)^2/3)^2 - 1))/100 + (3*(tanh(log((10*dt)/3)^2/3 - log(1 - (10*dt)/3)^2/3)^2 - 1)*((20*dt)/3 + tanh(((2^(1/2)*(log((10*dt)/3) + log(2 - (10*dt)/3)))/2 - 1)*(log((10*dt)/3) - log(2 - (10*dt)/3))) - 1)*((2*log((10*dt)/3))/(3*dt^2) - (200*log(1 - (10*dt)/3))/(27*((10*dt)/3 - 1)^2) + 200/(27*((10*dt)/3 - 1)^2) - 2/(3*dt^2)))/200 - (3*(tanh(((2^(1/2)*(log(1 - (10*dt)/3) + log((10*dt)/3 + 1)))/2 - 1)*(log(1 - (10*dt)/3) - log((10*dt)/3 + 1)))^2 - 1)*(tanh(log((10*dt)/3)^2/3 - log(1 - (10*dt)/3)^2/3)/2 - 1/2)*((100/(9*((10*dt)/3 - 1)^2) - 100/(9*((10*dt)/3 + 1)^2))*((2^(1/2)*(log(1 - (10*dt)/3) + log((10*dt)/3 + 1)))/2 - 1) - 2^(1/2)*(10/(3*((10*dt)/3 - 1)) - 10/(3*((10*dt)/3 + 1)))*(10/(3*((10*dt)/3 - 1)) + 10/(3*((10*dt)/3 + 1))) + (2^(1/2)*(100/(9*((10*dt)/3 - 1)^2) + 100/(9*((10*dt)/3 + 1)^2))*(log(1 - (10*dt)/3) - log((10*dt)/3 + 1)))/2))/100 - (3*tanh(((2^(1/2)*(log(1 - (10*dt)/3) + log((10*dt)/3 + 1)))/2 - 1)*(log(1 - (10*dt)/3) - log((10*dt)/3 + 1)))*(tanh(log((10*dt)/3)^2/3 - log(1 - (10*dt)/3)^2/3)^2 - 1)*((2*log((10*dt)/3))/(3*dt^2) - (200*log(1 - (10*dt)/3))/(27*((10*dt)/3 - 1)^2) + 200/(27*((10*dt)/3 - 1)^2) - 2/(3*dt^2)))/200 - (3*tanh(log((10*dt)/3)^2/3 - log(1 - (10*dt)/3)^2/3)*tanh(((2^(1/2)*(log(1 - (10*dt)/3) + log((10*dt)/3 + 1)))/2 - 1)*(log(1 - (10*dt)/3) - log((10*dt)/3 + 1)))*((2*log((10*dt)/3))/(3*dt) - (20*log(1 - (10*dt)/3))/(9*((10*dt)/3 - 1)))^2*(tanh(log((10*dt)/3)^2/3 - log(1 - (10*dt)/3)^2/3)^2 - 1))/100 - (3*tanh(((2^(1/2)*(log(1 - (10*dt)/3) + log((10*dt)/3 + 1)))/2 - 1)*(log(1 - (10*dt)/3) - log((10*dt)/3 + 1)))*(tanh(((2^(1/2)*(log(1 - (10*dt)/3) + log((10*dt)/3 + 1)))/2 - 1)*(log(1 - (10*dt)/3) - log((10*dt)/3 + 1)))^2 - 1)*((10/(3*((10*dt)/3 - 1)) - 10/(3*((10*dt)/3 + 1)))*((2^(1/2)*(log(1 - (10*dt)/3) + log((10*dt)/3 + 1)))/2 - 1) + (2^(1/2)*(10/(3*((10*dt)/3 - 1)) + 10/(3*((10*dt)/3 + 1)))*(log(1 - (10*dt)/3) - log((10*dt)/3 + 1)))/2)^2*(tanh(log((10*dt)/3)^2/3 - log(1 - (10*dt)/3)^2/3)/2 - 1/2))/50 + (3*tanh(log((10*dt)/3)^2/3 - log(1 - (10*dt)/3)^2/3)*((2*log((10*dt)/3))/(3*dt) - (20*log(1 - (10*dt)/3))/(9*((10*dt)/3 - 1)))^2*(tanh(log((10*dt)/3)^2/3 - log(1 - (10*dt)/3)^2/3)^2 - 1)*((20*dt)/3 + tanh(((2^(1/2)*(log((10*dt)/3) + log(2 - (10*dt)/3)))/2 - 1)*(log((10*dt)/3) - log(2 - (10*dt)/3))) - 1))/100 - (3*(tanh(((2^(1/2)*(log(1 - (10*dt)/3) + log((10*dt)/3 + 1)))/2 - 1)*(log(1 - (10*dt)/3) - log((10*dt)/3 + 1)))^2 - 1)*((2*log((10*dt)/3))/(3*dt) - (20*log(1 - (10*dt)/3))/(9*((10*dt)/3 - 1)))*((10/(3*((10*dt)/3 - 1)) - 10/(3*((10*dt)/3 + 1)))*((2^(1/2)*(log(1 - (10*dt)/3) + log((10*dt)/3 + 1)))/2 - 1) + (2^(1/2)*(10/(3*((10*dt)/3 - 1)) + 10/(3*((10*dt)/3 + 1)))*(log(1 - (10*dt)/3) - log((10*dt)/3 + 1)))/2)*(tanh(log((10*dt)/3)^2/3 - log(1 - (10*dt)/3)^2/3)^2 - 1))/100;

qv = [qd;dqd;ddqd]; %Send values back

end

function ris=compute_traj_parameters(s0, v0, sf, vm, am)
    ris=zeros(15,1);
    radix=zeros(2,1);
    T1 = 0;
    dT = 0;
    T2 = 0;
    a1 = 0;
    b1 = 0;
    c1 = 0;
    d1 = 0;
    e1 = 0;
    a2 = 0;
    b2 = 0;
    c2 = 0;
    d2 = 0;
    e2 = 0;
    k = 0;

    if (vm~=0) %check...
        vm=vm*sign(sf-s0);
        k=am*sign(sf-s0);
        T1 = -3/2*(v0-vm)/k;
        a1 = -4/27*k^3/(v0-vm)^2;
        b1 = -4/9*k^2/(v0-vm);
        e1 = s0;
        d1 = v0;
        c1 = 0;
        c2 = 0;
        T2 = 3/2*vm/k;
        dT = 1/4*(-3*vm^2+4*sf*k-4*a1*T1^4*k-4*b1*T1^3*k-4*c1*T1^2*k-4*d1*T1*k-4*e1*k)/vm/k;
        a2 = 4/27*k^3/vm^2;
        d2 = vm;
        e2 = 1/4*(-3*vm^2+4*sf*k)/k;
        b2 = -4/9*k^2/vm;
        if (dT<0)
            c2 = 0;
            c1 = 0;
            a=2;
            b=12*v0;
            c=9*v0^2-12*sf*k+12*s0*k;
            radix(1)=(-b + sqrt(b^2-4*a*c))/(2*a);
            radix(2)=(-b - sqrt(b^2-4*a*c))/(2*a);
            %decide the correct root
            T1_a = 1/2*radix(1)/k;
            T2_a = 1/2*(radix(1)+3*v0)/k;
            T1_b = 1/2*radix(2)/k;
            T2_b = 1/2*(radix(2)+3*v0)/k;
                if (and(T1_a>=0, T2_a>=0))
                    r=radix(1);
                    T1=T1_a;
                    T2=T2_a;
                    dT=0;
                    two_phases=1;
                elseif (and(T1_b>=0, T2_b>=0))
                    r=radix(2);
                    T1=T1_b;
                    T2=T2_b;
                    dT=0;
                    two_phases=1;
                else
                    r=0;
                    two_phases=0;
                end
                if (two_phases==0)
                    T1=0;
                    T2=2*(sf-s0)/v0;
                    dT=0;
                    b2=-1/4*v0^3/(sf-s0)^2;
                    c2=0;
                    a2=1/16*v0^4/(sf-s0)^3;
                    d2=v0;
                    e2=s0;
                else
                    b1 = -8/9*k^2/(4*v0*r+3*v0^2-4*sf*k+4*s0*k)*r;
                    a1 = 8/9*k^3/(4*v0*r+3*v0^2-4*sf*k+4*s0*k);
                    b2 = -8/9*k^2/(4*sf*k+3*v0^2-4*s0*k)*(r+3*v0);
                    e2 = -1/8*(3*v0^2-4*s0*k-4*sf*k)/k;
                    e1 = s0;
                    d1 = v0;
                    d2 = 2/9/(4*sf*k+3*v0^2-4*s0*k)*(r+3*v0)^3;
                    a2 = 8/9*k^3/(4*sf*k+3*v0^2-4*s0*k);
                end
        end
    end
    ris=[T1;dT;T2; a1; b1; c1; d1; e1; a2; b2; c2; d2; e2; vm; k];
end

%time, and the output of the previous function
function [ris, finished]=interpolator(t, parameters)

ris=zeros(3,1);
T1=parameters(1);
dT=parameters(2);
T2=parameters(3);
a1=parameters(4);
b1=parameters(5);
c1=parameters(6);
d1=parameters(7);
e1=parameters(8);
a2=parameters(9);
b2=parameters(10);
c2=parameters(11);
d2=parameters(12);
e2=parameters(13);
vm=parameters(14);
k=parameters(15);

finished = 0;
if (vm~=0) %check...
        if (t<=T1)
            ris=[a1*t^4+b1*t^3+c1*t^2+d1*t+e1; 4*a1*t^3+3*b1*t^2+2*c1*t+d1; 12*a1*t^2+6*b1*t+2*c1];
        elseif (t<=T1+dT)
            t=t-T1;
            ris=[a1*T1^4+b1*T1^3+c1*T1^2+d1*T1+e1+vm*t; vm; 0];
        elseif (t<=T1+dT+T2)
            t=t-T1-dT;
            ris=[a2*t^4+b2*t^3+c2*t^2+d2*t+e2; 4*a2*t^3+3*b2*t^2+2*c2*t+d2; 12*a2*t^2+6*b2*t+2*c2];
        else
            t=T2;
            ris=[a2*t^4+b2*t^3+c2*t^2+d2*t+e2;0;0];
            finished=1;
        end
else
    ris=[0;0;0];
end

end

function t=interpolator_1(q, parameters)

T1=parameters(1);
dT=parameters(2);
T2=parameters(3);
a1=parameters(4);
b1=parameters(5);
c1=parameters(6);
d1=parameters(7);
e1=parameters(8);
a2=parameters(9);
b2=parameters(10);
c2=parameters(11);
d2=parameters(12);
e2=parameters(13);
vm=parameters(14);
k=parameters(15);

t=0;
Q1 = a1*T1^4+b1*T1^3+c1*T1^2+d1*T1+e1;%q point at end of startup
Q2 = a2*T2^4+b2*T2^3+c2*T2^2+d2*T2+e2;%final q
Q3 = Q2-Q1;%q point at end of linear part (using symmetry)

if q<Q1
    %startup
%     %tarray = 0:0.001:T1; %not working, because T1 should be constant?!
%     tarray = linspace(0,T1);
%     qarray=zeros(size(tarray));
%     parfor i=1:size(tarray,2)
%         [qv,~]=interpolator(tarray(i), parameters);
%         qarray(i)=qv(1);
%     end
%     t = interp1(qarray, tarray, q);
    t=0;
    error('trans: interpolator_1 startup: not programmed jet, sry');
    % problem with calculating additional shift
elseif q>=Q1 || q<=Q3
    %linear part
    t = T1+((q-Q1)/vm);
elseif q>Q3
    %slowdown
    t=0;
    error('trans: interpolator_1 slowdown: not programmed jet, sry');
end

end
